simulink subsystem "log_ref"  (R2022a)
settings: Solver=VariableStepAuto  StartTime=0.0  StopTime=10.0  RelTol=1e-3
settings Model: Creator=tshintai  LastModifiedBy=tshintai

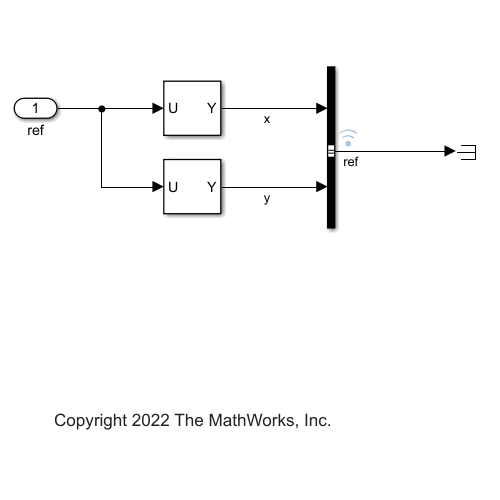
[thumbnail: Simulink's stored preview of the top-level diagram]
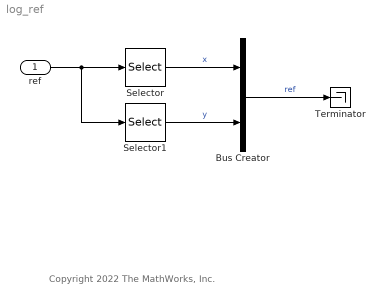
== system log_ref ==
  note: Copyright 2022 The MathWorks, Inc.
  ref : Inport
  Bus Creator : BusCreator  Inputs=2  OutDataTypeStr=Bus: Bus_pos
  Selector : Selector  NumberOfDimensions=2  InputPortWidth=3  IndexOptions=Index vector (dialog),Index vector (dialog)  Indices=1,1  OutputSizes=1,1
  Selector1 : Selector  NumberOfDimensions=2  InputPortWidth=3  IndexOptions=Index vector (dialog),Index vector (dialog)  Indices=2,1  OutputSizes=1,1
  Terminator : Terminator
  wires:
  ref/1 -> Selector/1, Selector1/1
  Selector/1 -> Bus Creator/1  "x"
  Selector1/1 -> Bus Creator/2  "y"
  Bus Creator/1 -> Terminator/1  "ref"
